simulink model "dc_mot_steady"  (R2019b)
settings: Solver=VariableStepAuto  StartTime=0.0  StopTime=400  RelTol=1e-3
InitFcn:
  | Ra = 1.2; % Armature resistance
  | La = 2.5e-3; %armature inductance
  | Kc = 0.35; %flux constant
  | J = 1e-3; % moment of inertia
  | %% Gains of the 2DOF PI current controller
  | alphac = 2*pi*500; %closed loop bandwidth
  | Kpc = alphac*La; % proportional gain
  | Kic = alphac*2*La; %integral gain
  | r = Kpc- Ra; %active resistance
  | Umax = 72; %saturation: upper limit
  | Umin = -72; %saturation lower limit
settings Model: Creator=srikesh  LastModifiedBy=srikesh

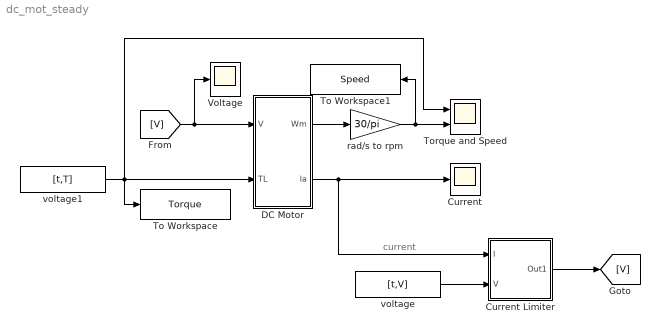
== system dc_mot_steady ==
  note: current
  Current : Scope
  Current Limiter : Subsystem
  "DC Motor " : Subsystem  mask{Ra=.1472, Ke=1.27, Kt=.9852}
      mask prompts: Ra "Ra(Ohm)"; Ke "Ke(V-s)"; Kt "Kt(N-m/A)"
  To Workspace : ToWorkspace  VariableName=Torque  SaveFormat=Timeseries  SampleTime=-1
  To Workspace1 : ToWorkspace  VariableName=Speed  SaveFormat=Timeseries  SampleTime=-1
  Torque and Speed : Scope  NumInputPorts=2
  Voltage : Scope
  "rad/s to rpm " : Gain  Gain=30/pi
  voltage : FromWorkspace  VariableName=[t,V]  SampleTime=0
  voltage1 : FromWorkspace  VariableName=[t,T]  SampleTime=0
  wires:
  voltage1/1 -> Torque and Speed/1, To Workspace/1, "DC Motor "/2("TL ")
  "DC Motor "/1("Wm ") -> "rad/s to rpm "/1
  [V] -> Voltage/1, "DC Motor "/1("V ")
  "DC Motor "/2(Ia) -> Current Limiter/1("I "), Current/1
  voltage/1 -> Current Limiter/2(V)
  Current Limiter/1(Out1) -> [V]
  "rad/s to rpm "/1 -> To Workspace1/1, Torque and Speed/2

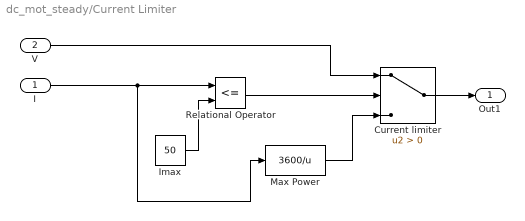
== system dc_mot_steady/Current Limiter ==
  "I " : Inport
  V : Inport  Port=2
  "Current limiter " : Switch  Criteria=u2 > Threshold
  Imax : Constant  Value=50
  Max Power : Fcn  Expr=3600/u
  Relational Operator : RelationalOperator  Operator=<=  OutDataTypeStr=boolean  RndMeth=Simplest
  Out1 : Outport
  wires:
  Max Power/1 -> "Current limiter "/3
  Imax/1 -> Relational Operator/2
  "I "/1 -> Relational Operator/1, Max Power/1
  V/1 -> "Current limiter "/1
  Relational Operator/1 -> "Current limiter "/2
  "Current limiter "/1 -> Out1/1

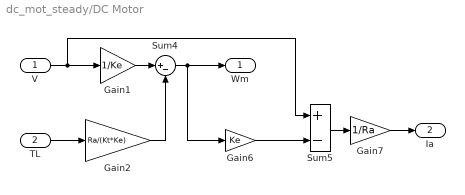
== system dc_mot_steady/DC Motor  ==
  "V " : Inport
  "TL " : Inport  Port=2
  Gain1 : Gain  Gain=1/Ke
  Gain2 : Gain  Gain=Ra/(Kt*Ke)
  Gain6 : Gain  Gain=Ke
  Gain7 : Gain  Gain=1/Ra
  Sum4 : Sum  Inputs=|+-
  Sum5 : Sum  Inputs=+-
  "Wm " : Outport
  Ia : Outport  Port=2
  wires:
  "V "/1 -> Sum5/1, Gain1/1
  Gain1/1 -> Sum4/1
  "TL "/1 -> Gain2/1
  Gain2/1 -> Sum4/2
  Sum4/1 -> Gain6/1, "Wm "/1
  Gain6/1 -> Sum5/2
  Gain7/1 -> Ia/1
  Sum5/1 -> Gain7/1
